simulink model "plant_test"  (R2025b)
settings: Solver=VariableStepAuto  StartTime=0.0  StopTime=10.0  RelTol=1e-3
undefined symbols (not defined in the file): p
settings Model: Creator=C4gie  LastModifiedBy=C4gie

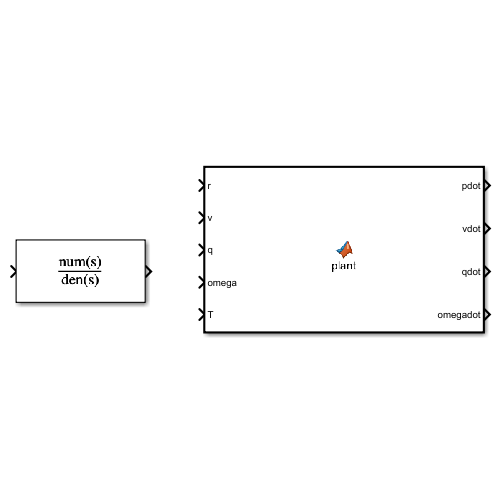
[thumbnail: Simulink's stored preview of the top-level diagram]
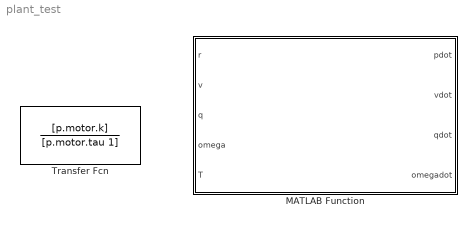
== system plant_test ==
  MATLAB Function : MATLAB Function  TreatAsAtomicUnit=on
  Transfer Fcn : TransferFcn  Numerator=[p.motor.k]  Denominator=[p.motor.tau 1]

== matlab function plant_test/MATLAB Function ==
  data: pdot output; r input; v input; q input; omega input; T input; vdot output; qdot output; omegadot output
function [pdot, vdot, qdot, omegadot] = plant(r, v, q, omega, T)
    [pdot, vdot, qdot, omegadot] = plant(r, v, q, omega, T);
end
